simulink model "IF_test"  (R2023b)
settings: Solver=VariableStepAuto  StartTime=0.0  StopTime=2  RelTol=1e-3
libraries: arduinolib x1, simulink x1
settings Model: Creator=FM22  LastModifiedBy=FM22

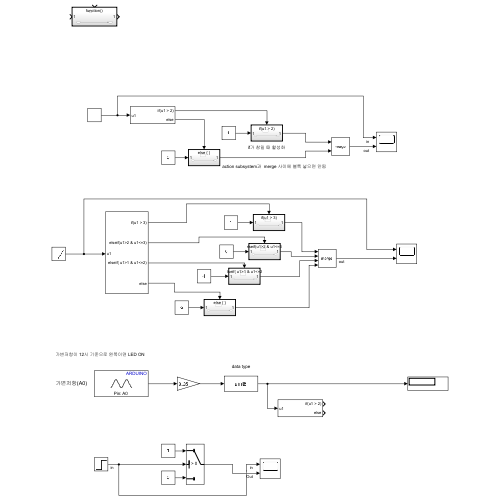
[thumbnail: Simulink's stored preview of the top-level diagram]
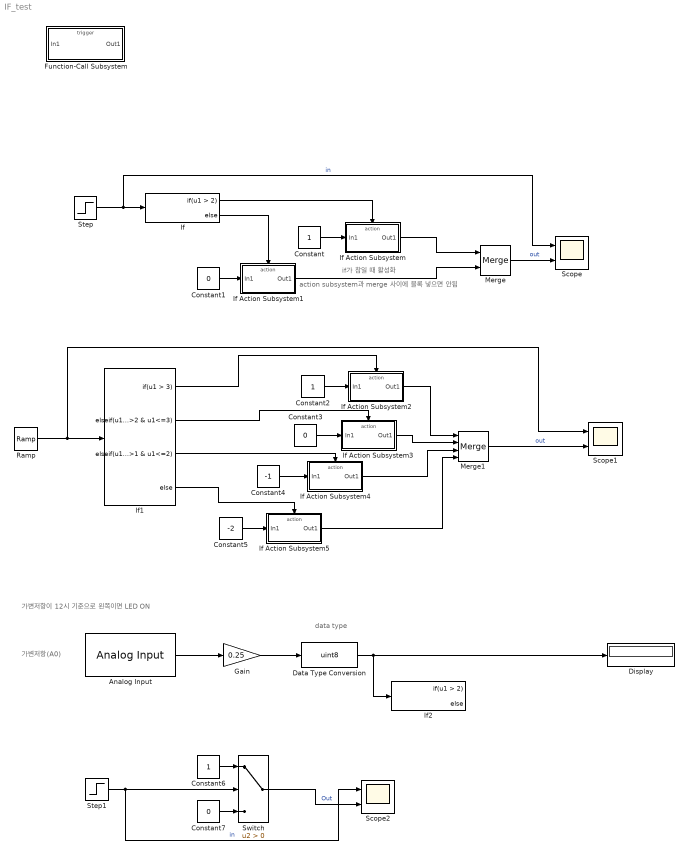
== system IF_test ==
  note: 가변저항이 12시 기준으로 왼쪽이면 LED ON
  note: if가 참일 때 활성화
  note: action subsystem과 merge 사이에 블록 넣으면 안됨
  note: data type
  note: 가변저항(A0)
  Analog Input : arduinolib/Analog Input  pinNumber=0  ReadResultsOnly=off  ConversionTriggerSource=Software  ExternalTriggerType=uint32( 0 )  OutputDataType=uint16  EnableConversionCompleteNotify=off  EnableOuputStatus=off  SampleTime=-1  blockPlatform=arduino
  Constant : Constant
  Constant1 : Constant  Value=0
  Constant2 : Constant
  Constant3 : Constant  Value=0
  Constant4 : Constant  Value=-1
  Constant5 : Constant  Value=-2
  Constant6 : Constant
  Constant7 : Constant  Value=0
  Data Type Conversion : DataTypeConversion  OutDataTypeStr=uint8  SaturateOnIntegerOverflow=off  RndMeth=Floor
  Display : Display
  Function-Call Subsystem : Subsystem  TreatAsAtomicUnit=on
  Gain : Gain  Gain=0.25
  If : If  IfExpression=u1 > 2
  If Action Subsystem : Subsystem  TreatAsAtomicUnit=on
  If Action Subsystem1 : Subsystem  TreatAsAtomicUnit=on
  If Action Subsystem2 : Subsystem  TreatAsAtomicUnit=on
  If Action Subsystem3 : Subsystem  TreatAsAtomicUnit=on
  If Action Subsystem4 : Subsystem  TreatAsAtomicUnit=on
  If Action Subsystem5 : Subsystem  TreatAsAtomicUnit=on
  If1 : If  IfExpression=u1 > 3  ElseIfExpressions=u1>2 & u1<=3, u1>1 & u1<=2
  If2 : If  IfExpression=u1 > 2
  Merge : Merge
  Merge1 : Merge  Inputs=4
  Ramp : simulink/Sources/Ramp  slope=1  start=0  InitialOutput=0
  Scope : Scope  NumInputPorts=2
  Scope1 : Scope  NumInputPorts=2
  Scope2 : Scope  NumInputPorts=2
  Step : Step  SampleTime=0
  Step1 : Step  SampleTime=0
  Switch : Switch  Criteria=u2 > Threshold  SaturateOnIntegerOverflow=off  InputSameDT=off
  wires:
  If/1 -> If Action Subsystem/Action
  Constant/1 -> If Action Subsystem/1(In1)
  Step/1 -> Scope/1, If/1  "in"
  If/2 -> If Action Subsystem1/Action
  Constant1/1 -> If Action Subsystem1/1(In1)
  If Action Subsystem1/1(Out1) -> Merge/2
  If Action Subsystem/1(Out1) -> Merge/1
  Merge/1 -> Scope/2  "out"
  Constant2/1 -> If Action Subsystem2/1(In1)
  Constant3/1 -> If Action Subsystem3/1(In1)
  Constant4/1 -> If Action Subsystem4/1(In1)
  Constant5/1 -> If Action Subsystem5/1(In1)
  If1/1 -> If Action Subsystem2/Action
  If1/2 -> If Action Subsystem3/Action
  If1/3 -> If Action Subsystem4/Action
  If1/4 -> If Action Subsystem5/Action
  Ramp/1 -> Scope1/1, If1/1
  Merge1/1 -> Scope1/2  "out"
  If Action Subsystem2/1(Out1) -> Merge1/1
  If Action Subsystem3/1(Out1) -> Merge1/2
  If Action Subsystem4/1(Out1) -> Merge1/3
  If Action Subsystem5/1(Out1) -> Merge1/4
  Data Type Conversion/1 -> If2/1, Display/1
  Gain/1 -> Data Type Conversion/1
  Analog Input/1 -> Gain/1
  Step1/1 -> Scope2/1, Switch/2  "in"
  Switch/1 -> Scope2/2  "Out"
  Constant6/1 -> Switch/1
  Constant7/1 -> Switch/3

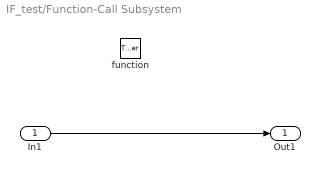
== system IF_test/Function-Call Subsystem ==
  In1 : Inport
  function : TriggerPort  TriggerType=function-call  VariantControl=(inherit)
  Out1 : Outport
  wires:
  In1/1 -> Out1/1

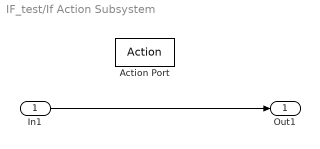
== system IF_test/If Action Subsystem ==
  In1 : Inport
  Action Port : ActionPort  ActionPortLabel=if(u1 > 2)
  Out1 : Outport
  wires:
  In1/1 -> Out1/1

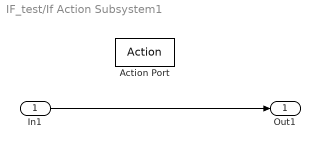
== system IF_test/If Action Subsystem1 ==
  In1 : Inport
  Action Port : ActionPort  ActionPortLabel=else
  Out1 : Outport
  wires:
  In1/1 -> Out1/1

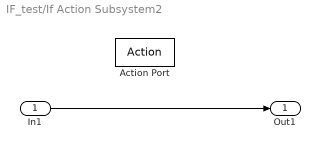
== system IF_test/If Action Subsystem2 ==
  In1 : Inport
  Action Port : ActionPort  ActionPortLabel=if(u1 > 3)
  Out1 : Outport
  wires:
  In1/1 -> Out1/1

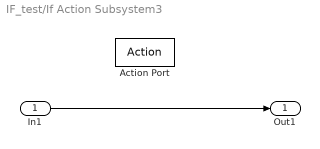
== system IF_test/If Action Subsystem3 ==
  In1 : Inport
  Action Port : ActionPort  ActionPortLabel=elseif(u1>2 & u1<=3)
  Out1 : Outport
  wires:
  In1/1 -> Out1/1

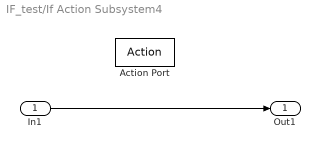
== system IF_test/If Action Subsystem4 ==
  In1 : Inport
  Action Port : ActionPort  ActionPortLabel=elseif( u1>1 & u1<=2)
  Out1 : Outport
  wires:
  In1/1 -> Out1/1

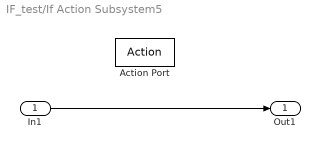
== system IF_test/If Action Subsystem5 ==
  In1 : Inport
  Action Port : ActionPort  ActionPortLabel=else
  Out1 : Outport
  wires:
  In1/1 -> Out1/1
